simulink model "Schema"  (R2020b)
settings: Solver=VariableStepAuto  StartTime=0.0  StopTime=50  RelTol=1e-3
undefined symbols (not defined in the file or in its folder): DELTA, G, Kx, Y
settings Model: Creator=teora  LastModifiedBy=teora

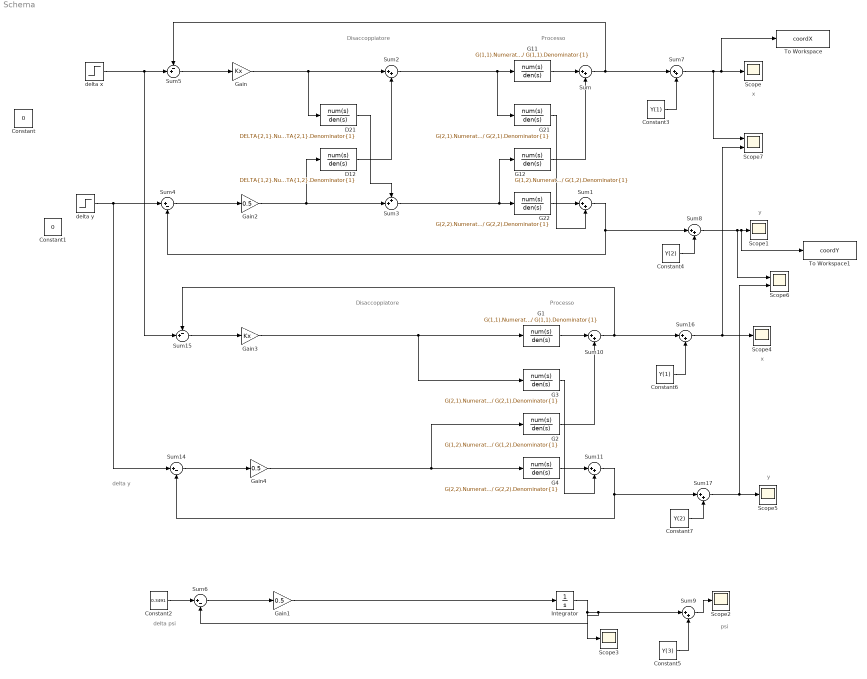
== system Schema ==
  note: delta psi
  note: psi
  note: y
  note: x
  note: Disaccoppiatore
  note: Processo
  note: y
  note: Processo
  note: x
  note: Disaccoppiatore
  note: delta y
  Constant : Constant  Value=0
  Constant1 : Constant  Value=0
  Constant2 : Constant  Value=0.3491
  Constant3 : Constant  Value=Y(1)
  Constant4 : Constant  Value=Y(2)
  Constant5 : Constant  Value=Y(3)
  Constant6 : Constant  Value=Y(1)
  Constant7 : Constant  Value=Y(2)
  D12 : TransferFcn  Numerator=DELTA{1,2}.Numerator{1}  Denominator=DELTA{1,2}.Denominator{1}
  D21 : TransferFcn  Numerator=DELTA{2,1}.Numerator{1}  Denominator=DELTA{2,1}.Denominator{1}
  G1 : TransferFcn  Numerator=G(1,1).Numerator{1}  Denominator=G(1,1).Denominator{1}
  G11 : TransferFcn  Numerator=G(1,1).Numerator{1}  Denominator=G(1,1).Denominator{1}
  G12 : TransferFcn  Numerator=G(1,2).Numerator{1}  Denominator=G(1,2).Denominator{1}
  G2 : TransferFcn  Numerator=G(1,2).Numerator{1}  Denominator=G(1,2).Denominator{1}
  G21 : TransferFcn  Numerator=G(2,1).Numerator{1}  Denominator=G(2,1).Denominator{1}
  G22 : TransferFcn  Numerator=G(2,2).Numerator{1}  Denominator=G(2,2).Denominator{1}
  G3 : TransferFcn  Numerator=G(2,1).Numerator{1}  Denominator=G(2,1).Denominator{1}
  G4 : TransferFcn  Numerator=G(2,2).Numerator{1}  Denominator=G(2,2).Denominator{1}
  Gain : Gain  Gain=Kx
  Gain1 : Gain  Gain=0.5
  Gain2 : Gain  Gain=0.5
  Gain3 : Gain  Gain=Kx
  Gain4 : Gain  Gain=0.5
  Integrator : Integrator
  Scope{,1..5} (6 alike) : Scope
  Scope6 : Scope  NumInputPorts=2
  Scope7 : Scope  NumInputPorts=2
  Sum{,1..2,7..11,16..17} (10 alike) : Sum  Inputs=|++
  Sum14 : Sum  Inputs=|+-
  Sum15 : Sum  Inputs=-+|
  Sum3 : Sum  Inputs=++|
  Sum4 : Sum  Inputs=|+-
  Sum5 : Sum  Inputs=-+|
  Sum6 : Sum  Inputs=|+-
  To Workspace : ToWorkspace  VariableName=coordX  SaveFormat=Timeseries  SampleTime=-1
  To Workspace1 : ToWorkspace  VariableName=coordY  SaveFormat=Timeseries  SampleTime=-1
  delta x : Step  Time=5  After=10  SampleTime=0
  delta y : Step  Time=5  After=50  SampleTime=0
  wires:
  G11/1 -> Sum/1
  G22/1 -> Sum1/1
  G12/1 -> Sum/2
  G21/1 -> Sum1/2
  D21/1 -> Sum3/1
  D12/1 -> Sum2/2
  Sum2/1 -> G21/1, G11/1
  Sum3/1 -> G12/1, G22/1
  Sum4/1 -> Gain2/1
  Sum1/1 -> Sum8/1, Sum4/2
  Sum/1 -> Sum7/1, Sum5/1
  Sum5/1 -> Gain/1
  Constant2/1 -> Sum6/1
  Sum6/1 -> Gain1/1
  Integrator/1 -> Scope3/1, Sum9/1, Sum6/2
  Constant3/1 -> Sum7/2
  Sum7/1 -> Scope7/1, To Workspace/1, Scope/1
  Constant4/1 -> Sum8/2
  Sum8/1 -> Scope6/1, To Workspace1/1, Scope1/1
  Constant5/1 -> Sum9/2
  Sum9/1 -> Scope2/1
  Gain/1 -> D21/1, Sum2/1
  Gain2/1 -> Sum3/2, D12/1
  Gain1/1 -> Integrator/1
  delta x/1 -> Sum15/2, Sum5/2
  Sum15/1 -> Gain3/1
  Constant6/1 -> Sum16/2
  Constant7/1 -> Sum17/2
  Sum17/1 -> Scope6/2, Scope5/1
  G4/1 -> Sum11/1
  G2/1 -> Sum10/2
  Sum14/1 -> Gain4/1
  G3/1 -> Sum11/2
  Sum11/1 -> Sum17/1, Sum14/2
  delta y/1 -> Sum14/1, Sum4/1
  G1/1 -> Sum10/1
  Sum16/1 -> Scope7/2, Scope4/1
  Sum10/1 -> Sum16/1, Sum15/1
  Gain3/1 -> G3/1, G1/1
  Gain4/1 -> G2/1, G4/1
